simulink model "exp5_beta_rootH"  (R2023a)
settings: Solver=VariableStepAuto  StartTime=0.0  StopTime=23  RelTol=1e-3
settings Model: Creator=nipun  LastModifiedBy=nipun

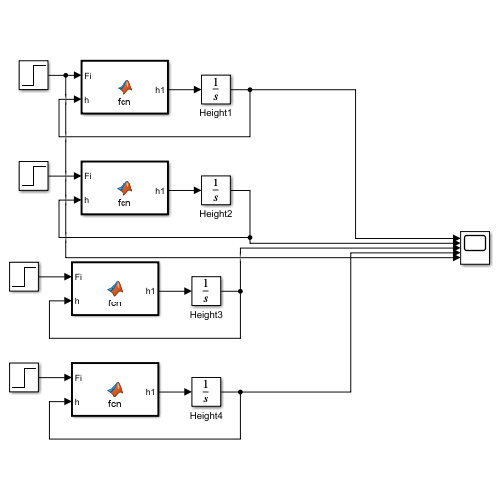
[thumbnail: Simulink's stored preview of the top-level diagram]
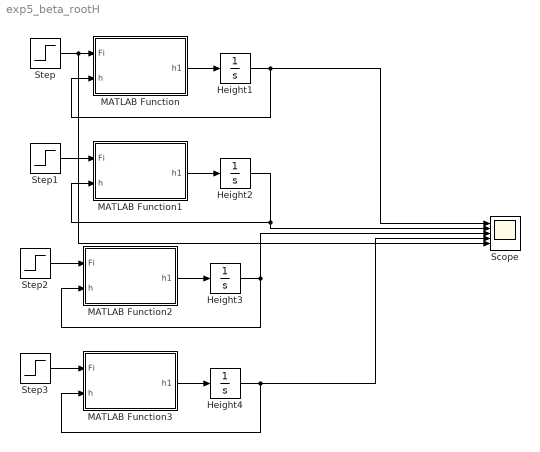
== system exp5_beta_rootH ==
  Height{1..4} (4 alike) : Integrator
  MATLAB Function : MATLAB Function  TreatAsAtomicUnit=on
  MATLAB Function1 : MATLAB Function  TreatAsAtomicUnit=on
  MATLAB Function2 : MATLAB Function  TreatAsAtomicUnit=on
  MATLAB Function3 : MATLAB Function  TreatAsAtomicUnit=on
  Scope : Scope  NumInputPorts=5
  Step{,1..3} (4 alike) : Step  Time=0  After=2  SampleTime=0
  wires:
  MATLAB Function/1(h1) -> Height1/1
  Height1/1 -> MATLAB Function/2(h), Scope/1
  Step/1 -> Scope/5, MATLAB Function/1(Fi)
  Step1/1 -> MATLAB Function1/1(Fi)
  Height2/1 -> Scope/2, MATLAB Function1/2(h)
  MATLAB Function1/1(h1) -> Height2/1
  MATLAB Function2/1(h1) -> Height3/1
  Height3/1 -> MATLAB Function2/2(h), Scope/3
  Step2/1 -> MATLAB Function2/1(Fi)
  Step3/1 -> MATLAB Function3/1(Fi)
  Height4/1 -> Scope/4, MATLAB Function3/2(h)
  MATLAB Function3/1(h1) -> Height4/1

== matlab function exp5_beta_rootH/MATLAB Function ==
  data: Fi input; h1 output; h input
function h1 = fcn(Fi,h)
ho=1;
A=1;
B=1;    
h1 = (Fi-(B*sqrt(ho)/2)-(B*h/(2*sqrt(ho))))/A;

== matlab function exp5_beta_rootH/MATLAB Function2 ==
  data: Fi input; h1 output; h input
function h1 = fcn(Fi,h)
ho=1;
A=1;
B=2;    
h1 = (Fi-B*sqrt(ho)/2-B*h/(2*sqrt(ho)))/A;

== matlab function exp5_beta_rootH/MATLAB Function3 ==
  data: Fi input; h1 output; h input
function h1 = fcn(Fi,h)
ho=4;
A=1;
B=1;    
h1 = (Fi-B*sqrt(ho)/2-B*h/(2*sqrt(ho)))/A;

== matlab function exp5_beta_rootH/MATLAB Function1 ==
  data: Fi input; h1 output; h input
function h1 = fcn(Fi,h)
ho=1;
A=2;
B=1;    
h1 = (Fi-B*sqrt(ho)/2-B*h/(2*sqrt(ho)))/A;
